simulink model "chap5_11sim"  (Simulink 7.7)
settings: Solver=ode45  StartTime=0.0  StopTime=20  RelTol=1e-3
settings Model: Creator=ljk  LastModifiedBy=ljk
settings DataIOCC: SignalLoggingName=sigsOut
settings DebuggingCC: SaveWithParameterizedLinksMsg=none  SignalResolutionControl=TryResolveAllWithWarning  SolverPrmCheckMsg=none  MultiTaskDSMMsg=warning  MultiTaskCondExecSysMsg=none  StrictBusMsg=None
settings HardwareCC: TargetUnknown=on
settings RTWCC: IncludeERTFirstTime=on

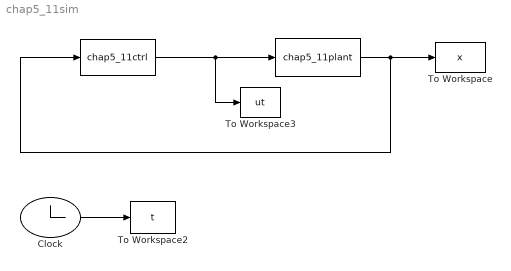
== system chap5_11sim ==
  "  " : S-Function  FunctionName=chap5_11plant  EnableBusSupport=off
  "    " : S-Function  FunctionName=chap5_11ctrl  EnableBusSupport=off
  Clock : Clock
      settings: Decimation=10
  To Workspace : ToWorkspace  VariableName=x  SampleTime=-1  SaveFormat=Array
  To Workspace2 : ToWorkspace  VariableName=t  SampleTime=-1  SaveFormat=Array
  To Workspace3 : ToWorkspace  VariableName=ut  SampleTime=-1  SaveFormat=Array
  wires:
  "  "/1 -> To Workspace/1, "    "/1
  "    "/1 -> To Workspace3/1, "  "/1
  Clock/1 -> To Workspace2/1
